simulink model "Joystick20140108"  (R2012b)
settings: Solver=ode4  StartTime=0.0  StopTime=inf  FixedStep=sample_time  RelTol=1e-3
InitFcn:
  | sample_time=0.005;%0.004;%0.0025;%0.02;
  | sample_time_Vicon = 0.005;
  | DeltaT = 0.02;
  | g = 9.81;
  | H0 = g%0.3165;
  | Kl = 1;
  | 
  | Omega_r = 1.31;%for Horizontal reference
  | Zeta_r = 1; %for Horizontal reference
  | Omega = 1.31;%for Horizontal Control
  | Zeta = 0.7;    %for Horizontal Control
  | 
  | Omega_h_r = 2.2; %for vertical reference
  | Zeta_h_r = 1;  %for vertical reference
  | Omega_h = 2.2;    %for vertical control
  | Zeta_h = 1;         %for vertical control
  | PI=pi;
  | 
  | Mass = 1.1;
  | Acc_Max = 4;
  | Acc_Max_h = 4;
  | 
  | Max_RP = 60;
  | 
  | % for NN
  | n = 5;
  | r = 3;
  | n2 = 5;
  | NN_ST = 0.02;
  | 
  | GAMA_V = 3;
  | gama_V_e = 0.01;
  | 
  | GAMA_W = GAMA_V;
  | gama_W_e =0.01;
  | 
  | % deadzone
  | NN_Deadzone_Z = 0;
  | 
  | % inputs nomalizaton parameters
  | NN_Z_y_min = -3;
  | NN_Z_y_max = 0.5;
  | 
  | NN_Z_v_max = 8;
  | NN_Z_v_min = -NN_Z_v_max;
  | 
  | % alpha = 0.034;
  | alpha = 1;
  | % c_f = 0.0015;
  | c_f = 0.001;
  | c_y_tilt = 1*0.5;
  | 
  | %for WK paras
  | Heightcontrol = 0.08;
  | Scale_Factor=1;
  | yoffset=0;
  | 
  | load MaoBi_Oct04_2_int.mat
  | MB_Interp.time = [];
undefined symbols (not defined in the file or in its folder): DiscIntNeverNeededParam
libraries: simulink x12, X330_Control x4, vrlib x1
(part 2 of 2)

== system Joystick20140108/Vicon_Data/Raw Quad Pose from Vicon/Process Vicon Raw Data6/Flip_pi1/Flip_0_to_2pi/Flip_2pi ==
  Angle : Inport
  Bias : Bias  Bias=-2*pi
  Constant : Constant  Value=2*pi
  Data Type Duplicate : DataTypeDuplicate
  Modulo : Math  Operator=mod  SaturateOnIntegerOverflow=on
  Sign1 : Signum
  Switch : Switch
  Angle_Flip : Outport
  wires:
  Angle/1 -> Modulo/1, Sign1/1, Data Type Duplicate/1
  Constant/1 -> Modulo/2
  Modulo/1 -> Bias/1, Switch/1
  Sign1/1 -> Switch/2
  Bias/1 -> Switch/3
  Switch/1 -> Angle_Flip/1, Data Type Duplicate/2

== system Joystick20140108/Vicon_Data/Raw Quad Pose from Vicon/Process Vicon Raw Data7/Flip_pi1/Flip_0_to_2pi/Flip_2pi ==
  Angle : Inport
  Bias : Bias  Bias=-2*pi
  Constant : Constant  Value=2*pi
  Data Type Duplicate : DataTypeDuplicate
  Modulo : Math  Operator=mod  SaturateOnIntegerOverflow=on
  Sign1 : Signum
  Switch : Switch
  Angle_Flip : Outport
  wires:
  Switch/1 -> Data Type Duplicate/2, Angle_Flip/1
  Bias/1 -> Switch/3
  Sign1/1 -> Switch/2
  Modulo/1 -> Switch/1, Bias/1
  Constant/1 -> Modulo/2
  Angle/1 -> Data Type Duplicate/1, Sign1/1, Modulo/1

== matlab function Joystick20140108/Joystick Mapping/check if quad are too close1 ==
  data: JoyReset input; u input; ClawPWM output; counter data_store_memory; PWMclaw data_store_memory; JOYtrigger output; clawdone input double size=1
function [ClawPWM, JOYtrigger] = CLAW(JoyReset, u, clawdone)
global counter;
global PWMclaw;


if(JoyReset==1)
    ClawPWM = PWMclaw;
    JOYtrigger = u;

else

    if(clawdone==2)
        PWMclaw = 1200;
        ClawPWM = PWMclaw;
        JOYtrigger = u;
        
    elseif(clawdone==3)
        PWMclaw = 1690;
        ClawPWM = PWMclaw;
        JOYtrigger = u;
    
    elseif(u~=1)
        if(PWMclaw==1690)
            counter = 1;
            ClawPWM = PWMclaw; 
            JOYtrigger = u;
        elseif (PWMclaw==1200)
            counter = 0;
            ClawPWM = PWMclaw;
            JOYtrigger = u;
        end
    

    
    else
        if(counter==1)
            PWMclaw = 1200;
            ClawPWM = PWMclaw;
            JOYtrigger = u;
        elseif(counter==0)
            PWMclaw = 1690;
            ClawPWM = PWMclaw;
            JOYtrigger = u;
        end
    
    end

    ClawPWM = PWMclaw;
    JOYtrigger = u;
    
end
   
end

== stateflow chart Joystick20140108/Planning/Trajectory Logic/UAV SF ==
  state AirBorne
    state Game
      state DecendPick
        state OutZone
          state ResetJoyDecent
            du:PosDesired [2]	= (-0.98-PosDesired[2])*0.3*DeltaT + PosDesired[2];
          state Resumeback
            en: ClawDone = 1;
          state CloseClaw
            en:
            PWM = 1200;
            ClawDone = 2;
          state ResetJoy
            en: JoystickReset	= 1;
          state Ascent
            du:
            PosDesired [2]	= (Joystick[2]-PosDesired[2])*0.01*DeltaT + PosDesired[2];
          (default) -> ResetJoyDecent : {PWM 			= 1690;
              | LightPWM		= 1750;}
          ResetJoyDecent -> CloseClaw : [abs(Pos[2]+0.98)<0.03]
          ResetJoy -> Resumeback
          CloseClaw -> Ascent : after (1,sec)
          Ascent -> ResetJoy : [abs(Pos[2]-PosDesired[2])<0.03]
        state InZone
          state MovetoCenter
            en:
            PosDesired [0]	= 0;
            PosDesired [1]	= 0;
          state Descent3
            du:PosDesired [2]	= (-0.98-PosDesired[2])*0.3*DeltaT + PosDesired[2];
          state Resumeback2
            en: ClawDone = 1;
          state ResetJoy1
            en: JoystickReset	= 1;
          state CloseClaw1
            en:
            PWM = 1200;
            ClawDone =2;
          state Ascent1
            du:
            PosDesired [2]	 = (Joystick[2]-PosDesired[2])*0.01*DeltaT + PosDesired[2];
          state Descent
            en:PosDesired [2] = -0.86;
          (default) -> Descent3 : {PWM			= 1690;
              | LightPWM		= 1650;}
          Descent3 -> MovetoCenter : [abs(Pos[2]+0.98)<0.03]
          MovetoCenter -> Descent : [(abs(Pos[0]-PosDesired[0])+abs(Pos[1]-PosDesired[1]))<0.015]
          ResetJoy1 -> Resumeback2
          Ascent1 -> ResetJoy1 : [abs(Pos[2]-PosDesired[2])<0.03]
          CloseClaw1 -> Ascent1 : after (1,sec)
          Descent -> CloseClaw1 : [abs(Pos[2]-PosDesired [2])<0.01]
        (default) -> (junction 1387)
        (junction 1387) -> OutZone [order 2] : [(TooClose[1]<=0.65)&&(TooClose[1]>=0.4)]
        (junction 1387) -> InZone [order 1] : [(TooClose[1]<0.4)]
      state JoystickCon
        du: PosDesired [0]  	= Joystick[0];
        PosDesired [1]	= Joystick[1];
        PosDesired [2]  	= Joystick[2];
        PWM 			= Joystick[3];
        LightPWM		= 1450;
      state ResetJoyStick1
        en:
        JoystickReset	= 0;
      state Fly
        du:
        PosDesired[0] = (XFly-PosDesired[0])*1.8*DeltaT + PosDesired[0];
        PosDesired[1] = (YFly-PosDesired[1])*1.8*DeltaT + PosDesired[1];
      state Flyaway
        en:
        XFly 			= TooClose[2];
        YFly 			= TooClose[3];
        JoystickReset 	= 1;
        LightPWM 		= 1250;
      DecendPick -> ResetJoyStick1 : [ClawDone ==1]
      JoystickCon -> DecendPick [order 1] : [(TooClose[1]<=0.45)&&(JoystickTrigger==1)]
      (default) -> ResetJoyStick1
      ResetJoyStick1 -> JoystickCon
      (junction 1449) -> ResetJoyStick1 [order 2] : [TooClose[0]==0]
      JoystickCon -> Flyaway [order 2] : [TooClose[0]==1]
      Fly -> (junction 1449) : after (2.5,sec)
      Flyaway -> Fly
      (junction 1449) -> Flyaway [order 1] : [TooClose[0]==1]
    state TakeOff
      du:HoverThrottle = (H0 - HoverThrottle)*3*DeltaT + HoverThrottle ;
      PosDesired[2]  = (-1.2- PosDesired[2])*1*DeltaT + PosDesired[2] ;
    state ResetJoyStick
      en:
      JoystickReset = 1;
      PosDesired [3] = 0;
    state Safety
      state HoverXY
        en:
        PosDesired 	= Pos;
        PWM 			= 1690;
        LightPWM 		= 1550;
      state HoverZ
        du:PosDesired[2] = (-1-PosDesired[2])*2*DeltaT + PosDesired[2];
      state OffloadPos
        du:
        PosDesired[0] = (0-PosDesired[0])*0.2*DeltaT + PosDesired[0];
        PosDesired[1] = (3.3-PosDesired[1])*0.2*DeltaT + PosDesired[1];
      state Descent2
        du: PosDesired[2] = (-0.57-PosDesired[2])*3*DeltaT + PosDesired[2];
      (default) -> HoverXY
      HoverXY -> HoverZ : [Q4[2]<-2]
      HoverZ -> OffloadPos : [abs(Pos[2]+1)<0.02]
      OffloadPos -> Descent2 : [(abs(Pos[0])+abs(Pos[1]-3.3))<0.3]
    note: Joystick[x]:
        |
        | 0. X-axis
        | 1. Y-axis
        | 2. Z-Axis
        | 3. PWM
        |
        | Joystick Trigger = Trigger state
        |
        |
        | TooClose[x]:
        |
        | Where x=:
        | 0.	Bound
        | 1.	Q5 Current Radius
        | 2.	X
        | 3.	Y
    (default) -> TakeOff : {PosDesired = Pos;}
    TakeOff -> ResetJoyStick : after (2.5,sec)
    ResetJoyStick -> Game
    Game -> Safety : [RC[5] > 0]
  state Landing
    state Descending
      en:PosDesired = Pos;
      du:PosDesired[2] = (0.2- PosDesired[2])*0.5*DeltaT + PosDesired[2] ;
    state CutThrottle
      en: PWM=1600;
      du:HoverThrottle = (0.0- HoverThrottle)*3*DeltaT + HoverThrottle ;
    (default) -> Descending : {LightPWM = 1550;}
    Descending -> CutThrottle : [Pos[2] >(0.0 -0.2)]
  (default) -> ? [order 1] : [(abs(Q4[0]+2)+abs(Q4[1]))<0.2]
  Landing -> AirBorne : [RC[6] > 0.5]
  AirBorne -> Landing : [RC[6] < -0.5]
  (default) -> Landing [order 1] : {HoverThrottle = 0;}
  data: PosDesired output double size=4; HoverThrottle output double size=1; LightPWM output uint16 size=1; RC input size=8; Pos input size=4; PerchPos input size=4; DeltaT parameter size=1; H0 parameter size=1; Kl parameter size=1; VelCmd local double size=2 =0; PWM output double; PerchError input; PI parameter size=1; descentrate local double; Joystick input; TooClose input double; JoystickReset output double size=1; XFly local double size=1; YFly local double size=1; ClawDone output double size=1; JoystickTrigger input boolean size=1; Q4 input

== matlab function Joystick20140108/Planning/check if quad are too close ==
  data: Q1 input; Q2 input; Q3 input; Q4 input; Q5 input; BOUND output; Q5CR output; XJoy output [-3.5..3.5]; YJoy output [-3.5..3.5]; PlatformAngle data_store_memory; XJoyOut data_store_memory; YJoyOut data_store_memory; XJoyIn data_store_memory; YJoyIn data_store_memory; TangentialAngle data_store_memory
function [BOUND, Q5CR,  XJoy, YJoy]   = Distance(Q1, Q2, Q3, Q4, Q5)

%  XJoyXInHalf, YJoyYInHalf, XTangentialInHalf, YTangentialInHalf,  XTangentialOutHalf, YTangentialOutHalf, XJoyXOutHalf, YJoyYOutHalf


global PlatformAngle;
global XJoyIn;
global YJoyIn;
global XJoyOut;
global YJoyOut;
global TangentialAngle;

%Distance between Joystick Quad and Formation Quad.
DQ1 = sqrt((Q5(1)-Q1(1))^2 + (Q5(2)-Q1(2))^2);
DQ2 = sqrt((Q5(1)-Q2(1))^2 + (Q5(2)-Q2(2))^2);
DQ3 = sqrt((Q5(1)-Q3(1))^2 + (Q5(2)-Q3(2))^2);
DQ4 = sqrt((Q5(1)-Q4(1))^2 + (Q5(2)-Q4(2))^2);

%Joystick quad current distance away from platform.


% PlatformAngle = atan2((Q5(2)-Platform(2)),(Q5(1)-Platform(1)));
PlatformAngle = atan2((Q5(1)),(Q5(2)));

%Coordinates to fly outwards while remaining 3m radius away from platform.

XJoyOut     = 3.4*sin(PlatformAngle);
YJoyOut     = 3.4*cos(PlatformAngle);

XJoyIn      = 0.5*sin(PlatformAngle);
YJoyIn      = 0.5*cos(PlatformAngle);

    
if ((DQ1<1.28)||(DQ2<1.28)||(DQ3<1.28)||(DQ4<1.28))
    
    BOUND       = 1;
    Q5CR        = sqrt(Q5(1)^2 + Q5(2)^2);
      
   if(Q5CR<1.75)
        XJoy    = XJoyIn;
        YJoy    = YJoyIn;
   
   elseif ((Q5CR>=1.75)&&(Q5CR<=2.35))    
        TangentialAngle = acos((sqrt(Q5(1)^2 + Q5(2)^2))/3.3);
        XJoy    = YJoyOut*sin(TangentialAngle) + XJoyOut*cos(TangentialAngle);
        YJoy    = YJoyOut*cos(TangentialAngle) - XJoyOut*sin(TangentialAngle);  
      
   else
        XJoy    = XJoyOut;
        YJoy    = YJoyOut;
       
    end
    
       

else
    
    BOUND       = 0;
    Q5CR        = sqrt(Q5(1)^2 + Q5(2)^2);
    
    if(Q5CR<2)
        XJoy    = XJoyIn;
        YJoy    = YJoyIn;
     
   else
        XJoy    = XJoyOut;
        YJoy    = YJoyOut;       
       
    end

end
end
